simulink library "Matrix4x4"  (Simulink 6.2)
settings Model: LastModifiedBy=rolf

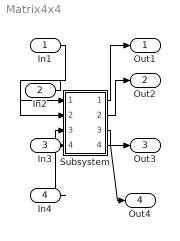
== system Matrix4x4 ==
  In1 : Inport  Port=1  LatchInput=off
  In2 : Inport  Port=2  LatchInput=off
  In3 : Inport  Port=3  LatchInput=off
  In4 : Inport  Port=4  LatchInput=off
  Subsystem : Subsystem
  Out1 : Outport
  Out2 : Outport  Port=2
  Out3 : Outport  Port=3
  Out4 : Outport  Port=4
  wires:
  Subsystem/1(Out1) -> Out1/1
  In1/1 -> Subsystem/1(In1)
  Subsystem/2(Out2) -> Out2/1
  In2/1 -> Subsystem/2(In2)
  Subsystem/3(Out3) -> Out3/1
  In3/1 -> Subsystem/3(In3)
  In4/1 -> Subsystem/4(In4)
  Subsystem/4(Out4) -> Out4/1

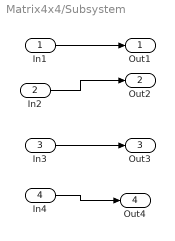
== system Matrix4x4/Subsystem ==
  In1 : Inport  Port=1  LatchInput=off
  In2 : Inport  Port=2  LatchInput=off
  In3 : Inport  Port=3  LatchInput=off
  In4 : Inport  Port=4  LatchInput=off
  Out1 : Outport
  Out2 : Outport  Port=2
  Out3 : Outport  Port=3
  Out4 : Outport  Port=4
  wires:
  In4/1 -> Out4/1
  In3/1 -> Out3/1
  In2/1 -> Out2/1
  In1/1 -> Out1/1
